simulink model "Modal_Control_Closed_Integ"  (R2018b)
settings: Solver=VariableStepAuto  StartTime=0.0  StopTime=200  RelTol=1e-3
values from neighbouring files (symbols this model uses):
  alpha = 0.5736    [constants.m]
  c_damp = 0.00495    [constants.m]
  in_nu = 0.0001    [constants.m]
  J_r = 0.0004    [constants.m]
  J_s = 31.38    [constants.m]
  time_cons = 0.5    [constants.m]
  w_mode = 2.6268    [constants.m]
settings Model: Creator=Yavuz  LastModifiedBy=Yavuz
settings DebuggingCC: AlgebraicLoopMsg=none

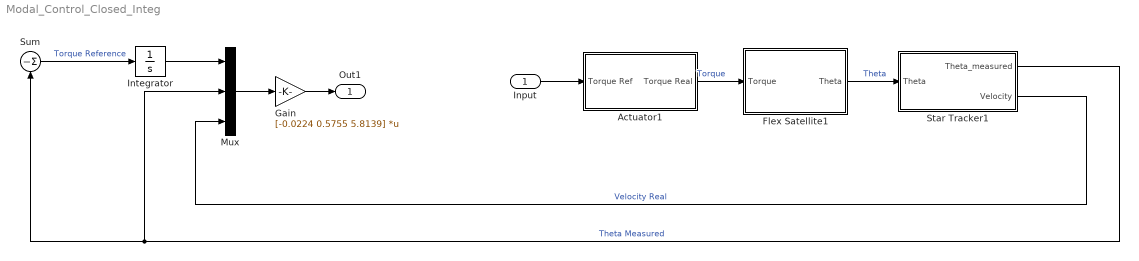
== system Modal_Control_Closed_Integ ==
  Input : Inport
  Actuator1 : Subsystem
  Flex Satellite1 : Subsystem
  Gain : Gain  Gain=[-0.0224 0.5755 5.8139]  Multiplication=Matrix(K*u)
  Integrator : Integrator
  Mux : Mux  Inputs=3
  Star Tracker1 : Subsystem
  Sum : Sum  Inputs=|-
  Out1 : Outport
  wires:
  Sum/1 -> Integrator/1  "Torque Reference"
  Integrator/1 -> Mux/1
  Actuator1/1(Torque Real) -> Flex Satellite1/1(Torque)  "Torque"
  Input/1 -> Actuator1/1(Torque Ref)
  Flex Satellite1/1(Theta) -> Star Tracker1/1(Theta)  "Theta"
  Star Tracker1/1(Theta_measured) -> Mux/2, Sum/1  "Theta Measured"
  Star Tracker1/2(Velocity) -> Mux/3  "Velocity Real"
  Mux/1 -> Gain/1
  Gain/1 -> Out1/1

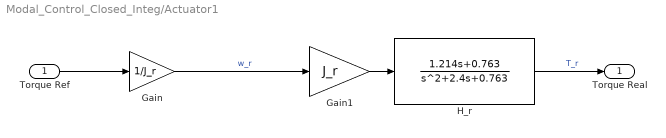
== system Modal_Control_Closed_Integ/Actuator1 ==
  Torque Ref : Inport
  Gain : Gain  Gain=1/J_r
  Gain1 : Gain  Gain=J_r
  H_r : TransferFcn  Numerator=[1.214 0.763]  Denominator=[1 2.4 0.763]
  Torque Real : Outport
  wires:
  Gain1/1 -> H_r/1
  H_r/1 -> Torque Real/1  "T_r"
  Torque Ref/1 -> Gain/1
  Gain/1 -> Gain1/1  "w_r"

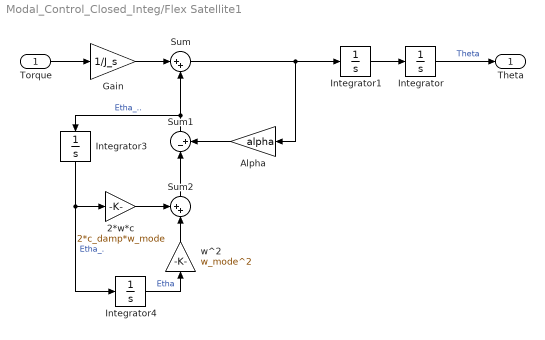
== system Modal_Control_Closed_Integ/Flex Satellite1 ==
  Torque : Inport
  2*w*c : Gain  Gain=2*c_damp*w_mode
  Alpha : Gain  Gain=alpha
  Gain : Gain  Gain=1/J_s
  Integrator : Integrator
  Integrator1 : Integrator
  Integrator3 : Integrator
  Integrator4 : Integrator  InitialCondition=in_nu
  Sum : Sum  Inputs=|++
  Sum1 : Sum  Inputs=|-+
  Sum2 : Sum  Inputs=++|
  w^2 : Gain  Gain=w_mode^2
  Theta : Outport
  wires:
  Sum/1 -> Integrator1/1, Alpha/1
  Sum1/1 -> Integrator3/1, Sum/2  "Etha_.."
  Gain/1 -> Sum/1
  Integrator1/1 -> Integrator/1
  Integrator3/1 -> Integrator4/1, 2*w*c/1  "Etha_."
  Sum2/1 -> Sum1/1
  Torque/1 -> Gain/1
  2*w*c/1 -> Sum2/1
  Integrator/1 -> Theta/1  "Theta"
  w^2/1 -> Sum2/2
  Integrator4/1 -> w^2/1  "Etha"
  Alpha/1 -> Sum1/2

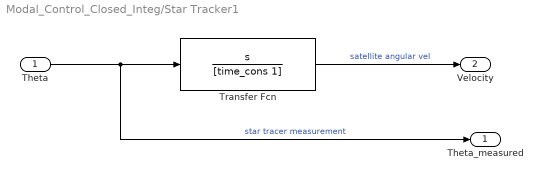
== system Modal_Control_Closed_Integ/Star Tracker1 ==
  Theta : Inport
  Transfer Fcn : TransferFcn  Numerator=[1 0]  Denominator=[time_cons 1]
  Theta_measured : Outport
  Velocity : Outport  Port=2
  wires:
  Theta/1 -> Theta_measured/1, Transfer Fcn/1  "star tracer measurement"
  Transfer Fcn/1 -> Velocity/1  "satellite angular vel"
